simulink model "simplifiedBicycleContinuousKinematic"  (R2018b)
settings: Solver=VariableStepAuto  StartTime=0.0  StopTime=50  RelTol=1e-3
libraries: simulink x1
settings Model: Creator=jasprit  LastModifiedBy=jasprit

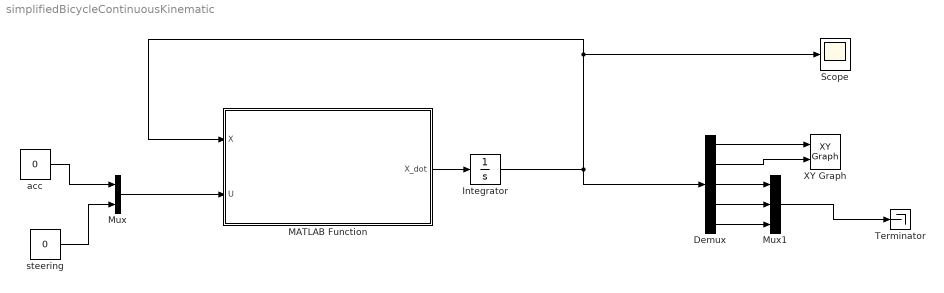
== system simplifiedBicycleContinuousKinematic ==
  Demux : Demux  Outputs=5
  Integrator : Integrator  InitialCondition=[0;0;0;10;0.05]
  MATLAB Function : MATLAB Function  TreatAsAtomicUnit=on
  Mux : Mux  Inputs=2
  Mux1 : Mux  Inputs=3
  Scope : Scope
  Terminator : Terminator
  XY Graph : simulink/Sinks/XY Graph  xmin=-200  xmax=200  ymin=-200  ymax=200  st=-1
  acc : Constant  Value=0
  steering : Constant  Value=0
  wires:
  steering/1 -> Mux/2
  acc/1 -> Mux/1
  Mux/1 -> MATLAB Function/2(U)
  MATLAB Function/1(X_dot) -> Integrator/1
  Demux/1 -> XY Graph/1
  Demux/2 -> XY Graph/2
  Mux1/1 -> Terminator/1
  Demux/3 -> Mux1/1
  Demux/4 -> Mux1/2
  Demux/5 -> Mux1/3
  Integrator/1 -> Demux/1, MATLAB Function/1(X), Scope/1

== matlab function simplifiedBicycleContinuousKinematic/MATLAB Function ==
  data: X input; X_dot output; U input
function X_dot = simplifiedKinematicBicycleModel(X, U)

    
    vehicle = SedanBicycleModelParameters();
    l = vehicle.l_r + vehicle.l_f;
    
    x = X(1);
    y = X(2);
    psi = X(3);
    v = X(4);
    delta = X(5);
    X_dot = [ v*cos(psi);
                v*sin(psi);
                v*tan(delta)/l;
                U(1);
                U(2)];
end
